simulink model "controller_test_2006a"  (Simulink 6.4)
settings: Solver=ode4  StartTime=0.0  StopTime=50  FixedStep=0.01  RelTol=1e-3
undefined symbols (not defined in the file or in its folder): DiscIntNeverNeededParam, trajectory_time
libraries: simulink x1
settings Model: Creator=Bazs  LastModifiedBy=Developer
settings OptimizationCC: InitFltsAndDblsToZero=off
settings DebuggingCC: SignalResolutionControl=UseLocalSettings  MultiTaskDSMMsg=error  MultiTaskCondExecSysMsg=error  FcnCallInpInsideContextMsg=Enable All  StrictBusMsg=ErrorLevel1
settings HardwareCC: TargetHWDeviceType=32-bit Generic
settings GRTTargetCC: CombineOutputUpdateFcns=on

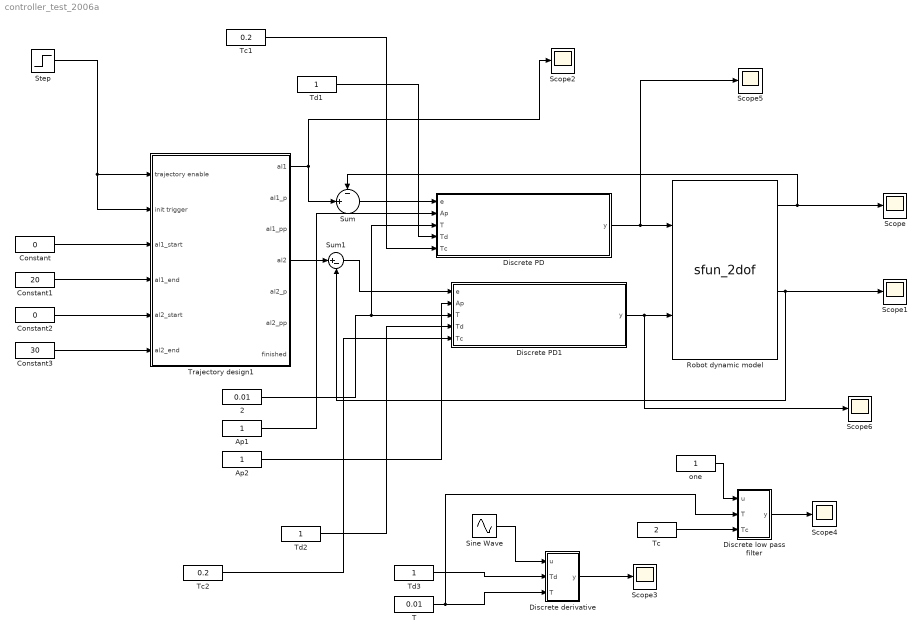
== system controller_test_2006a ==
  2 : Constant  Value=0.01  OutDataType=fixdt(1,16,0)  ConRadixGroup=Use specified scaling  OutScaling=[]  SampleTime=inf  FramePeriod=inf
  Ap1 : Constant  Value=1  OutDataType=fixdt(1,16,0)  ConRadixGroup=Use specified scaling  OutScaling=[]  SampleTime=inf  FramePeriod=inf
  Ap2 : Constant  Value=1  OutDataType=fixdt(1,16,0)  ConRadixGroup=Use specified scaling  OutScaling=[]  SampleTime=inf  FramePeriod=inf
  Constant : Constant  Value=0  OutDataType=fixdt(1,16,0)  ConRadixGroup=Use specified scaling  OutScaling=[]  SampleTime=inf  FramePeriod=inf
  Constant1 : Constant  Value=20  OutDataType=fixdt(1,16,0)  ConRadixGroup=Use specified scaling  OutScaling=[]  SampleTime=inf  FramePeriod=inf
  Constant2 : Constant  Value=0  OutDataType=fixdt(1,16,0)  ConRadixGroup=Use specified scaling  OutScaling=[]  SampleTime=inf  FramePeriod=inf
  Constant3 : Constant  Value=30  OutDataType=fixdt(1,16,0)  ConRadixGroup=Use specified scaling  OutScaling=[]  SampleTime=inf  FramePeriod=inf
  Discrete PD : Subsystem
  Discrete PD1 : Subsystem
  Discrete derivative : Subsystem
  Discrete low pass filter : Subsystem
  Robot dynamic model : M-S-Function  FunctionName=sfun_2dof  Parameters=0.4, 1, 0.2, 0.5, 0.2, 0.1
  Scope{,1..6} (7 alike) : Scope
      Scope settings: YMin=14  YMax=24
      Scope1 settings: TimeRange=50  YMin=0  YMax=35
      Scope2 settings: YMin=0  YMax=22.5  SaveName=ScopeData2
      Scope3 settings: YMin=-1  YMax=1  SaveName=ScopeData3
      Scope4 settings: YMin=0.98  YMax=1  SaveName=ScopeData4
      Scope5 settings: YMin=-2.5e-07  YMax=6.5e-07  SaveName=ScopeData6
      Scope6 settings: TimeRange=100  YMin=28.5  YMax=31.5  SaveName=ScopeData7
  Sine Wave : Sin  SampleTime=0
  Step : Step  Time=0.01  SampleTime=0
  Sum : Sum  Inputs=-|+||  OutDataType=fixdt(1,16,0)  OutScaling=[]
  Sum1 : Sum  Inputs=|+-  OutDataType=fixdt(1,16,0)  OutScaling=[]
  T : Constant  Value=0.01  OutDataType=fixdt(1,16,0)  ConRadixGroup=Use specified scaling  OutScaling=[]  SampleTime=inf  FramePeriod=inf
  Tc : Constant  Value=2  OutDataType=fixdt(1,16,0)  ConRadixGroup=Use specified scaling  OutScaling=[]  SampleTime=inf  FramePeriod=inf
  Tc1 : Constant  Value=0.2  OutDataType=fixdt(1,16,0)  ConRadixGroup=Use specified scaling  OutScaling=[]  SampleTime=inf  FramePeriod=inf
  Tc2 : Constant  Value=0.2  OutDataType=fixdt(1,16,0)  ConRadixGroup=Use specified scaling  OutScaling=[]  SampleTime=inf  FramePeriod=inf
  Td1 : Constant  Value=1  OutDataType=fixdt(1,16,0)  ConRadixGroup=Use specified scaling  OutScaling=[]  SampleTime=inf  FramePeriod=inf
  Td2 : Constant  Value=1  OutDataType=fixdt(1,16,0)  ConRadixGroup=Use specified scaling  OutScaling=[]  SampleTime=inf  FramePeriod=inf
  Td3 : Constant  Value=1  OutDataType=fixdt(1,16,0)  ConRadixGroup=Use specified scaling  OutScaling=[]  SampleTime=inf  FramePeriod=inf
  Trajectory design1 : Subsystem
  one : Constant  Value=1  OutDataType=fixdt(1,16,0)  ConRadixGroup=Use specified scaling  OutScaling=[]  SampleTime=inf  FramePeriod=inf
  wires:
  Discrete PD/1(y) -> Scope5/1, Robot dynamic model/1
  Discrete PD1/1(y) -> Scope6/1, Robot dynamic model/2
  Step/1 -> Trajectory design1/1(trajectory enable), Trajectory design1/2(init trigger)
  Constant/1 -> Trajectory design1/3(al1_start)
  Constant1/1 -> Trajectory design1/4(al1_end)
  Constant2/1 -> Trajectory design1/5(al2_start)
  Constant3/1 -> Trajectory design1/6(al2_end)
  Trajectory design1/1(al1) -> Sum/2, Scope2/1
  Robot dynamic model/1 -> Sum/1, Scope/1
  Trajectory design1/4(al2) -> Sum1/1
  Robot dynamic model/3 -> Sum1/2, Scope1/1
  Sum/1 -> Discrete PD/1(e)
  Sum1/1 -> Discrete PD1/1(e)
  Ap1/1 -> Discrete PD/2(Ap)
  Ap2/1 -> Discrete PD1/2(Ap)
  2/1 -> Discrete PD/3(T), Discrete PD1/3(T)
  Td1/1 -> Discrete PD/4(Td)
  Td2/1 -> Discrete PD1/4(Td)
  Tc1/1 -> Discrete PD/5(Tc)
  Tc2/1 -> Discrete PD1/5(Tc)
  Sine Wave/1 -> Discrete derivative/1(u)
  Td3/1 -> Discrete derivative/2(Td)
  T/1 -> Discrete derivative/3(T), Discrete low pass filter/2(T)
  Discrete derivative/1(y) -> Scope3/1
  Tc/1 -> Discrete low pass filter/3(Tc)
  one/1 -> Discrete low pass filter/1(u)
  Discrete low pass filter/1(y) -> Scope4/1

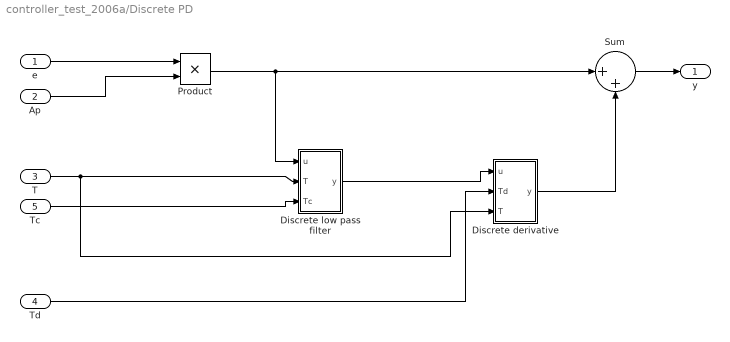
== system controller_test_2006a/Discrete PD ==
  e : Inport  OutDataType=fixdt(1,16,0)  OutScaling=[]
  Ap : Inport  Port=2  OutDataType=fixdt(1,16,0)  OutScaling=[]
  T : Inport  Port=3  OutDataType=fixdt(1,16,0)  OutScaling=[]
  Td : Inport  Port=4  OutDataType=fixdt(1,16,0)  OutScaling=[]
  Tc : Inport  Port=5  OutDataType=fixdt(1,16,0)  OutScaling=[]
  Discrete derivative : Subsystem
  Discrete low pass filter : Subsystem
  Product : Product  OutDataType=fixdt(1,16,0)  OutScaling=[]  RndMeth=Zero
  Sum : Sum  Inputs=|++  OutDataType=fixdt(1,16,0)  OutScaling=[]
  y : Outport  OutDataType=fixdt(1,16,0)  OutScaling=[]
  wires:
  Product/1 -> Discrete low pass filter/1(u), Sum/1
  e/1 -> Product/1
  Sum/1 -> y/1
  Ap/1 -> Product/2
  T/1 -> Discrete low pass filter/2(T), Discrete derivative/3(T)
  Tc/1 -> Discrete low pass filter/3(Tc)
  Td/1 -> Discrete derivative/2(Td)
  Discrete derivative/1(y) -> Sum/2
  Discrete low pass filter/1(y) -> Discrete derivative/1(u)

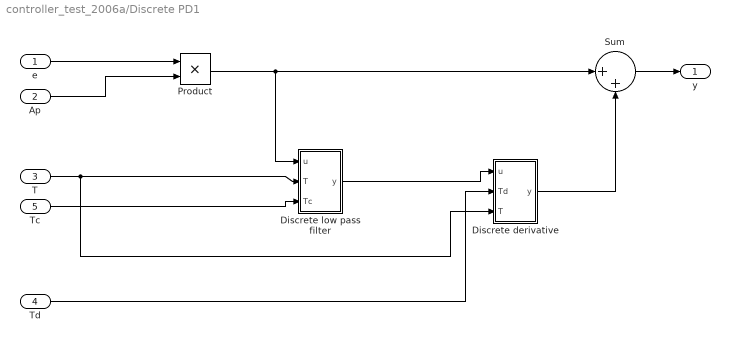
== system controller_test_2006a/Discrete PD1 ==
  e : Inport  OutDataType=fixdt(1,16,0)  OutScaling=[]
  Ap : Inport  Port=2  OutDataType=fixdt(1,16,0)  OutScaling=[]
  T : Inport  Port=3  OutDataType=fixdt(1,16,0)  OutScaling=[]
  Td : Inport  Port=4  OutDataType=fixdt(1,16,0)  OutScaling=[]
  Tc : Inport  Port=5  OutDataType=fixdt(1,16,0)  OutScaling=[]
  Discrete derivative : Subsystem
  Discrete low pass filter : Subsystem
  Product : Product  OutDataType=fixdt(1,16,0)  OutScaling=[]  RndMeth=Zero
  Sum : Sum  Inputs=|++  OutDataType=fixdt(1,16,0)  OutScaling=[]
  y : Outport  OutDataType=fixdt(1,16,0)  OutScaling=[]
  wires:
  Product/1 -> Discrete low pass filter/1(u), Sum/1
  e/1 -> Product/1
  Sum/1 -> y/1
  Ap/1 -> Product/2
  T/1 -> Discrete low pass filter/2(T), Discrete derivative/3(T)
  Tc/1 -> Discrete low pass filter/3(Tc)
  Td/1 -> Discrete derivative/2(Td)
  Discrete derivative/1(y) -> Sum/2
  Discrete low pass filter/1(y) -> Discrete derivative/1(u)

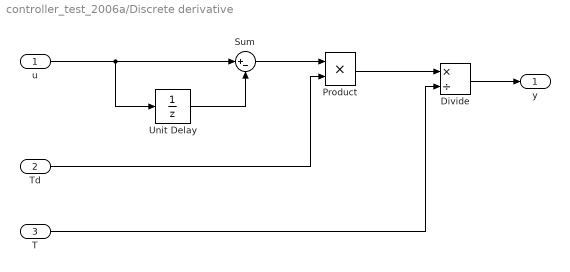
== system controller_test_2006a/Discrete derivative ==
  u : Inport  OutDataType=fixdt(1,16,0)  OutScaling=[]
  Td : Inport  Port=2  OutDataType=fixdt(1,16,0)  OutScaling=[]
  T : Inport  Port=3  OutDataType=fixdt(1,16,0)  OutScaling=[]
  Divide : Product  Inputs=*/  OutScaling=2^-10
  Product : Product  RndMeth=Zero
  Sum : Sum  Inputs=|+-
  Unit Delay : UnitDelay  SampleTime=-1
  y : Outport  OutDataType=fixdt(1,16,0)  OutScaling=[]
  wires:
  u/1 -> Unit Delay/1, Sum/1
  Unit Delay/1 -> Sum/2
  Sum/1 -> Product/1
  Td/1 -> Product/2
  Product/1 -> Divide/1
  T/1 -> Divide/2
  Divide/1 -> y/1

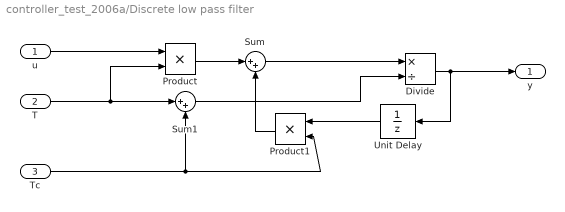
== system controller_test_2006a/Discrete low pass filter ==
  u : Inport  OutDataType=fixdt(1,16,0)  OutScaling=[]
  T : Inport  Port=2  OutDataType=fixdt(1,16,0)  OutScaling=[]
  Tc : Inport  Port=3  OutDataType=fixdt(1,16,0)  OutScaling=[]
  Divide : Product  Inputs=*/  OutScaling=2^-10
  Product : Product  RndMeth=Zero
  Product1 : Product  Orientation=left  RndMeth=Zero
  Sum : Sum  Inputs=|++
  Sum1 : Sum  Inputs=|++
  Unit Delay : UnitDelay  Orientation=left  SampleTime=-1
  y : Outport  OutDataType=fixdt(1,16,0)  OutScaling=[]
  wires:
  u/1 -> Product/1
  T/1 -> Product/2, Sum1/1
  Unit Delay/1 -> Product1/1
  Tc/1 -> Product1/2, Sum1/2
  Product/1 -> Sum/1
  Product1/1 -> Sum/2
  Sum/1 -> Divide/1
  Sum1/1 -> Divide/2
  Divide/1 -> Unit Delay/1, y/1

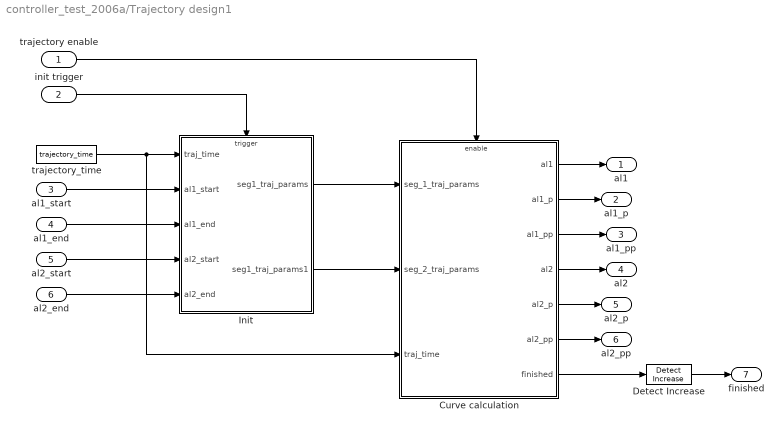
== system controller_test_2006a/Trajectory design1 ==
  trajectory enable : Inport  OutDataType=fixdt(1,16,0)  OutScaling=[]
  init trigger : Inport  Port=2  OutDataType=fixdt(1,16,0)  OutScaling=[]
  al1_start : Inport  Port=3  OutDataType=fixdt(1,16,0)  OutScaling=[]
  al1_end : Inport  Port=4  OutDataType=fixdt(1,16,0)  OutScaling=[]
  al2_start : Inport  Port=5  OutDataType=fixdt(1,16,0)  OutScaling=[]
  al2_end : Inport  Port=6  OutDataType=fixdt(1,16,0)  OutScaling=[]
  Curve calculation : Subsystem
  Detect Increase : simulink/Logic and Bit Operations/Detect Increase  SystemSampleTime=-1  vinit=0.0
  Init : Subsystem
  trajectory_time : Constant  Value=trajectory_time  OutDataType=fixdt(1,16,0)  ConRadixGroup=Use specified scaling  OutScaling=[]  SampleTime=inf  FramePeriod=inf
  al1 : Outport  OutDataType=fixdt(1,16,0)  OutScaling=[]
  al1_p : Outport  Port=2  OutDataType=fixdt(1,16,0)  OutScaling=[]
  al1_pp : Outport  Port=3  OutDataType=fixdt(1,16,0)  OutScaling=[]
  al2 : Outport  Port=4  OutDataType=fixdt(1,16,0)  OutScaling=[]
  al2_p : Outport  Port=5  OutDataType=fixdt(1,16,0)  OutScaling=[]
  al2_pp : Outport  Port=6  OutDataType=fixdt(1,16,0)  OutScaling=[]
  finished : Outport  Port=7  OutDataType=fixdt(1,16,0)  OutScaling=[]
  wires:
  trajectory_time/1 -> Curve calculation/3(traj_time), Init/1(traj_time)
  al1_end/1 -> Init/3(al1_end)
  Init/2(seg1_traj_params1) -> Curve calculation/2(seg_2_traj_params)
  Init/1(seg1_traj_params) -> Curve calculation/1(seg_1_traj_params)
  trajectory enable/1 -> Curve calculation/Enable
  Curve calculation/1(al1) -> al1/1
  Curve calculation/2(al1_p) -> al1_p/1
  al1_start/1 -> Init/2(al1_start)
  Curve calculation/3(al1_pp) -> al1_pp/1
  Curve calculation/4(al2) -> al2/1
  Curve calculation/5(al2_p) -> al2_p/1
  Curve calculation/6(al2_pp) -> al2_pp/1
  al2_start/1 -> Init/4(al2_start)
  al2_end/1 -> Init/5(al2_end)
  init trigger/1 -> Init/Trigger
  Curve calculation/7(finished) -> Detect Increase/1
  Detect Increase/1 -> finished/1

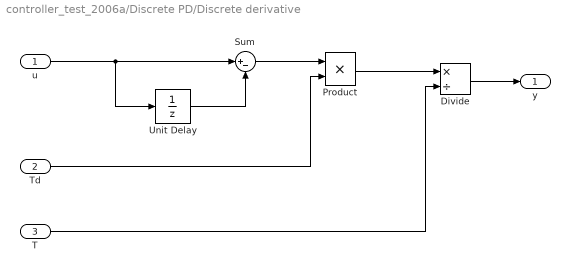
== system controller_test_2006a/Discrete PD/Discrete derivative ==
  u : Inport  OutDataType=fixdt(1,16,0)  OutScaling=[]
  Td : Inport  Port=2  OutDataType=fixdt(1,16,0)  OutScaling=[]
  T : Inport  Port=3  OutDataType=fixdt(1,16,0)  OutScaling=[]
  Divide : Product  Inputs=*/  OutScaling=2^-10
  Product : Product  RndMeth=Zero
  Sum : Sum  Inputs=|+-
  Unit Delay : UnitDelay  SampleTime=-1
  y : Outport  OutDataType=fixdt(1,16,0)  OutScaling=[]
  wires:
  u/1 -> Unit Delay/1, Sum/1
  Unit Delay/1 -> Sum/2
  Sum/1 -> Product/1
  Td/1 -> Product/2
  Product/1 -> Divide/1
  T/1 -> Divide/2
  Divide/1 -> y/1

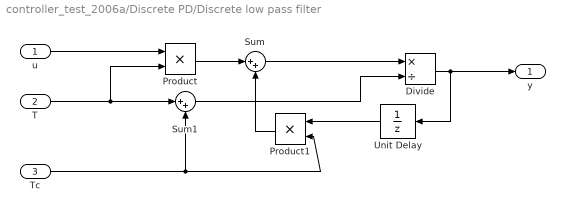
== system controller_test_2006a/Discrete PD/Discrete low pass filter ==
  u : Inport  OutDataType=fixdt(1,16,0)  OutScaling=[]
  T : Inport  Port=2  OutDataType=fixdt(1,16,0)  OutScaling=[]
  Tc : Inport  Port=3  OutDataType=fixdt(1,16,0)  OutScaling=[]
  Divide : Product  Inputs=*/  OutScaling=2^-10
  Product : Product  RndMeth=Zero
  Product1 : Product  Orientation=left  RndMeth=Zero
  Sum : Sum  Inputs=|++
  Sum1 : Sum  Inputs=|++
  Unit Delay : UnitDelay  Orientation=left  SampleTime=-1
  y : Outport  OutDataType=fixdt(1,16,0)  OutScaling=[]
  wires:
  u/1 -> Product/1
  T/1 -> Product/2, Sum1/1
  Unit Delay/1 -> Product1/1
  Tc/1 -> Product1/2, Sum1/2
  Product/1 -> Sum/1
  Product1/1 -> Sum/2
  Sum/1 -> Divide/1
  Sum1/1 -> Divide/2
  Divide/1 -> Unit Delay/1, y/1

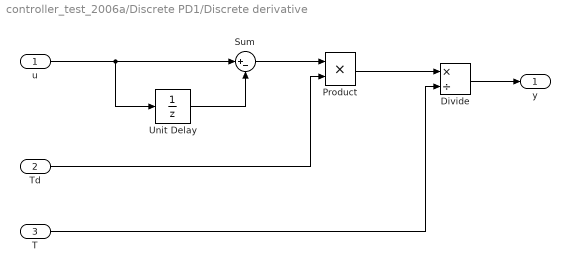
== system controller_test_2006a/Discrete PD1/Discrete derivative ==
  u : Inport  OutDataType=fixdt(1,16,0)  OutScaling=[]
  Td : Inport  Port=2  OutDataType=fixdt(1,16,0)  OutScaling=[]
  T : Inport  Port=3  OutDataType=fixdt(1,16,0)  OutScaling=[]
  Divide : Product  Inputs=*/  OutScaling=2^-10
  Product : Product  RndMeth=Zero
  Sum : Sum  Inputs=|+-
  Unit Delay : UnitDelay  SampleTime=-1
  y : Outport  OutDataType=fixdt(1,16,0)  OutScaling=[]
  wires:
  u/1 -> Unit Delay/1, Sum/1
  Unit Delay/1 -> Sum/2
  Sum/1 -> Product/1
  Td/1 -> Product/2
  Product/1 -> Divide/1
  T/1 -> Divide/2
  Divide/1 -> y/1

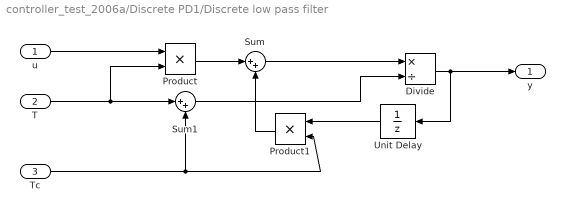
== system controller_test_2006a/Discrete PD1/Discrete low pass filter ==
  u : Inport  OutDataType=fixdt(1,16,0)  OutScaling=[]
  T : Inport  Port=2  OutDataType=fixdt(1,16,0)  OutScaling=[]
  Tc : Inport  Port=3  OutDataType=fixdt(1,16,0)  OutScaling=[]
  Divide : Product  Inputs=*/  OutScaling=2^-10
  Product : Product  RndMeth=Zero
  Product1 : Product  Orientation=left  RndMeth=Zero
  Sum : Sum  Inputs=|++
  Sum1 : Sum  Inputs=|++
  Unit Delay : UnitDelay  Orientation=left  SampleTime=-1
  y : Outport  OutDataType=fixdt(1,16,0)  OutScaling=[]
  wires:
  u/1 -> Product/1
  T/1 -> Product/2, Sum1/1
  Unit Delay/1 -> Product1/1
  Tc/1 -> Product1/2, Sum1/2
  Product/1 -> Sum/1
  Product1/1 -> Sum/2
  Sum/1 -> Divide/1
  Sum1/1 -> Divide/2
  Divide/1 -> Unit Delay/1, y/1

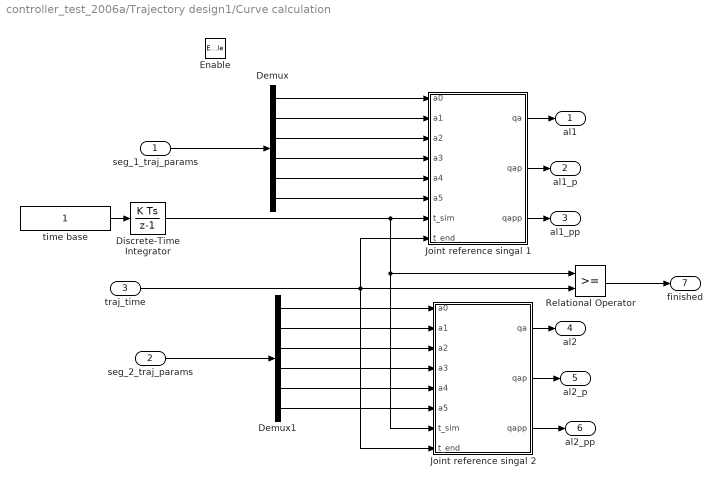
== system controller_test_2006a/Trajectory design1/Curve calculation ==
  seg_1_traj_params : Inport  OutDataType=fixdt(1,16,0)  OutScaling=[]
  seg_2_traj_params : Inport  Port=2  OutDataType=fixdt(1,16,0)  OutScaling=[]
  traj_time : Inport  Port=3  OutDataType=fixdt(1,16,0)  OutScaling=[]
  Enable : EnablePort  StatesWhenEnabling=reset
  Demux : Demux  Outputs=6
  Demux1 : Demux  Outputs=6
  Discrete-Time Integrator : DiscreteIntegrator  SampleTime=-1  OutDataType=fixdt(1,16,0)  OutScaling=[]  ICPrevOutput=DiscIntNeverNeededParam  ICPrevScaledInput=DiscIntNeverNeededParam
  Joint reference singal 1 : Stateflow chart  TreatAsAtomicUnit=on
  Joint reference singal 2 : Stateflow chart  TreatAsAtomicUnit=on
  Relational Operator : RelationalOperator  LogicOutDataTypeMode=Boolean
  time base : Constant  Value=1  OutDataType=fixdt(1,16,0)  ConRadixGroup=Use specified scaling  OutScaling=[]  SampleTime=inf  FramePeriod=inf
  al1 : Outport  OutDataType=fixdt(1,16,0)  OutScaling=[]
  al1_p : Outport  Port=2  OutDataType=fixdt(1,16,0)  OutScaling=[]
  al1_pp : Outport  Port=3  OutDataType=fixdt(1,16,0)  OutScaling=[]
  al2 : Outport  Port=4  OutDataType=fixdt(1,16,0)  OutScaling=[]
  al2_p : Outport  Port=5  OutDataType=fixdt(1,16,0)  OutScaling=[]
  al2_pp : Outport  Port=6  OutDataType=fixdt(1,16,0)  OutScaling=[]
  finished : Outport  Port=7  OutDataType=fixdt(1,16,0)  OutScaling=[]
  wires:
  Joint reference singal 1/1(qa) -> al1/1
  Joint reference singal 1/2(qap) -> al1_p/1
  Joint reference singal 1/3(qapp) -> al1_pp/1
  Joint reference singal 2/1(qa) -> al2/1
  Discrete-Time Integrator/1 -> Joint reference singal 1/7(t_sim), Joint reference singal 2/7(t_sim), Relational Operator/1
  time base/1 -> Discrete-Time Integrator/1
  Demux/1 -> Joint reference singal 1/1(a0)
  Demux/2 -> Joint reference singal 1/2(a1)
  Demux/3 -> Joint reference singal 1/3(a2)
  Demux/4 -> Joint reference singal 1/4(a3)
  Demux/5 -> Joint reference singal 1/5(a4)
  Demux/6 -> Joint reference singal 1/6(a5)
  Demux1/1 -> Joint reference singal 2/1(a0)
  Demux1/2 -> Joint reference singal 2/2(a1)
  Demux1/3 -> Joint reference singal 2/3(a2)
  Demux1/4 -> Joint reference singal 2/4(a3)
  Demux1/5 -> Joint reference singal 2/5(a4)
  Demux1/6 -> Joint reference singal 2/6(a5)
  seg_1_traj_params/1 -> Demux/1
  seg_2_traj_params/1 -> Demux1/1
  traj_time/1 -> Joint reference singal 1/8(t_end), Joint reference singal 2/8(t_end), Relational Operator/2
  Relational Operator/1 -> finished/1
  Joint reference singal 2/2(qap) -> al2_p/1
  Joint reference singal 2/3(qapp) -> al2_pp/1

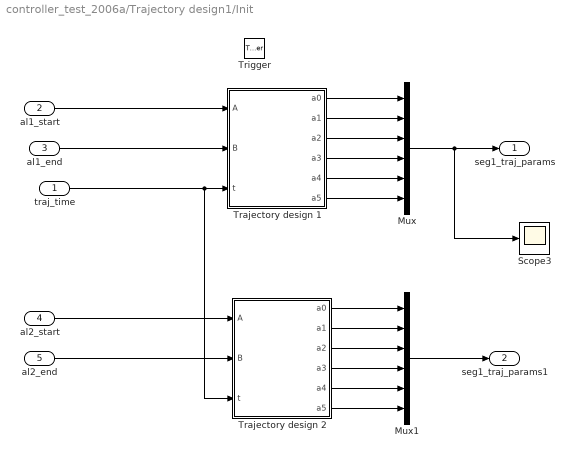
== system controller_test_2006a/Trajectory design1/Init ==
  traj_time : Inport  OutDataType=fixdt(1,16,0)  OutScaling=[]
  al1_start : Inport  Port=2  OutDataType=fixdt(1,16,0)  OutScaling=[]  LatchByDelayingOutsideSignal=on
  al1_end : Inport  Port=3  OutDataType=fixdt(1,16,0)  OutScaling=[]
  al2_start : Inport  Port=4  OutDataType=fixdt(1,16,0)  OutScaling=[]  LatchByDelayingOutsideSignal=on
  al2_end : Inport  Port=5  OutDataType=fixdt(1,16,0)  OutScaling=[]
  Trigger : TriggerPort
  Mux : Mux  Inputs=6
  Mux1 : Mux  Inputs=6
  Scope3 : Scope
      settings: YMin=38  YMax=42  SaveName=ScopeData5
  Trajectory design 1 : Stateflow chart  TreatAsAtomicUnit=on
  Trajectory design 2 : Stateflow chart  TreatAsAtomicUnit=on
  seg1_traj_params : Outport  OutDataType=fixdt(1,16,0)  OutScaling=[]
  seg1_traj_params1 : Outport  Port=2  OutDataType=fixdt(1,16,0)  OutScaling=[]
  wires:
  al1_start/1 -> Trajectory design 1/1(A)
  al1_end/1 -> Trajectory design 1/2(B)
  al2_start/1 -> Trajectory design 2/1(A)
  al2_end/1 -> Trajectory design 2/2(B)
  traj_time/1 -> Trajectory design 1/3(t), Trajectory design 2/3(t)
  Trajectory design 1/1(a0) -> Mux/1
  Trajectory design 1/2(a1) -> Mux/2
  Trajectory design 1/3(a2) -> Mux/3
  Trajectory design 1/4(a3) -> Mux/4
  Trajectory design 1/5(a4) -> Mux/5
  Trajectory design 1/6(a5) -> Mux/6
  Trajectory design 2/1(a0) -> Mux1/1
  Trajectory design 2/2(a1) -> Mux1/2
  Trajectory design 2/3(a2) -> Mux1/3
  Trajectory design 2/4(a3) -> Mux1/4
  Trajectory design 2/5(a4) -> Mux1/5
  Trajectory design 2/6(a5) -> Mux1/6
  Mux/1 -> seg1_traj_params/1, Scope3/1
  Mux1/1 -> seg1_traj_params1/1

== matlab function Trajectory design1/Curve calculation/Joint reference singal 1 ==
  data: a0 input double; a1 input double; a2 input double; a3 input double; a4 input double; a5 input double; t_sim input double; qa output double; qap output double; qapp output double; t_end input double
function [qa,qap,qapp] = fcn(a0,a1,a2,a3,a4,a5,t_sim,t_end)
% This block supports an embeddable subset of the MATLAB language.
% See the help menu for details. 
if (t_sim>=t_end) 
    t_sim = t_end;
end   
T = [t_sim^5/20 t_sim^4/12 t_sim^3/6 t_sim^2/2 t_sim 1;...
    t_sim^4/4 t_sim^3/3 t_sim^2/2 t_sim 1 0;...
    t_sim^3 t_sim^2 t_sim 1 0 0];
Q = T*[a0;a1;a2;a3;a4;a5];

qa = Q(1);
qap = Q(2);
qapp = Q(3);

== matlab function Trajectory design1/Curve calculation/Joint reference singal 2 ==
  data: a0 input double; a1 input double; a2 input double; a3 input double; a4 input double; a5 input double; t_sim input double; qa output double; qap output double; qapp output double; t_end input double
function [qa,qap,qapp] = fcn(a0,a1,a2,a3,a4,a5,t_sim,t_end)
% This block supports an embeddable subset of the MATLAB language.
% See the help menu for details. 
if (t_sim>=t_end) 
    t_sim = t_end;
end   
T = [t_sim^5/20 t_sim^4/12 t_sim^3/6 t_sim^2/2 t_sim 1;...
    t_sim^4/4 t_sim^3/3 t_sim^2/2 t_sim 1 0;...
    t_sim^3 t_sim^2 t_sim 1 0 0];
Q = T*[a0;a1;a2;a3;a4;a5];

qa = Q(1);
qap = Q(2);
qapp = Q(3);

== matlab function Trajectory design1/Init/Trajectory design 1 ==
  data: A input double; B input double; t input double; a0 output double; a1 output double; a2 output double; a3 output double; a4 output double; a5 output double
function [a0,a1,a2,a3,a4,a5] = fcn(A,B,t)
% This block supports an embeddable subset of the MATLAB language.
% See the help menu for details. 
T = [t^5/20 t^4/12 t^3/6 t^2/2 t 1;t^4/4 t^3/3 t^2/2 t 1 0;t^3 t^2 t 1 0 0;0 0 0 0 0 1;0 0 0 0 1 0;0 0 0 1 0 0];
Ao = inv(T)*[B;0;0;A;0;0];
a0=Ao(1);
a1=Ao(2);
a2=Ao(3);
a3=Ao(4);
a4=Ao(5);
a5=Ao(6);

== matlab function Trajectory design1/Init/Trajectory design 2 ==
  data: A input double; B input double; t input double; a0 output double; a1 output double; a2 output double; a3 output double; a4 output double; a5 output double
function [a0,a1,a2,a3,a4,a5] = fcn(A,B,t)
% This block supports an embeddable subset of the MATLAB language.
% See the help menu for details. 
T = [t^5/20 t^4/12 t^3/6 t^2/2 t 1;t^4/4 t^3/3 t^2/2 t 1 0;t^3 t^2 t 1 0 0;0 0 0 0 0 1;0 0 0 0 1 0;0 0 0 1 0 0];
Ao = inv(T)*[B;0;0;A;0;0];
a0=Ao(1);
a1=Ao(2);
a2=Ao(3);
a3=Ao(4);
a4=Ao(5);
a5=Ao(6);
